simulink model "AUV_ControlsPreliminary"  (R2020b)
settings: Solver=ode23t  StartTime=0.0  StopTime=300  MaxStep=0.01  RelTol=1e-3  EnableMultiTasking=on
PreLoadFcn:
  | AUV_VehicleParameters;
  | Vehicle.Body.markeropacity = 0;
model workspace: external: MATLAB File AUV_DataFile_ORIG.m (data not in the file)
undefined symbols (not defined in the file or in its folder): Environment, Newton, Raphson, smiData, X, x, y, Y, Z
libraries: sm_lib x3123, nesl_utility x51, sharedutil x8, pid_lib x6, AUVCustomPrimitives_Lib x4, shared6dof x1, aerolibasang x1, aerolibadyn x1, SignalEditorBlockLib x1
(part 1 of 62)
settings Model: Creator=cosorio  LastModifiedBy=cosorio
settings DataIOCC: MaxDataPoints=10000  SaveOutput=off  DSMLogging=off  SaveTime=off  SignalLoggingName=logsout_controls
settings OptimizationCC: LifeSpan=inf
settings DebuggingCC: AllowSymbolicDim=off  SFUnexpectedBacktrackingDiag=warning  SFNoUnconditionalDefaultTransitionDiag=warning  SFExecutionAtInitializationDiag=none  ArithmeticOperatorsInVariantConditions=warning
settings SFSimCC: SimUseLocalCustomCode=off  CustomCodeUndefinedFunction=UseInterfaceOnly
settings RTWCC: RTWUseLocalCustomCode=off
settings CodeAppCC: StateflowObjectComments=on
settings GRTTargetCC: TargetLangStandard=C89/C90 (ANSI)
settings ConfigComp: CovMetricSettings=dw  CovSaveCumulativeToWorkspaceVar=on  CovSaveSingleToWorkspaceVar=on  CovExternalEMLEnable=off  CovSFcnEnable=off
settings SimscapeCC: SimscapeLogName=simlog_hydrodynamicsVAR  SimscapeLogLimitData=off  SimscapeLogDataHistory=10000
settings DiagnosticsConfigSet: SimMechanicsUnconnectedFramePorts=none  SimMechanicsConflictingReferenceFrames=none
settings ExplorerConfigSet: InternalSimMechanicsExplorerSettings="<ExplorerConfiguration><canonicalview>aerospace</canonicalview><AnimationSetting><BasePlaybackSpeed>1.0</BasePlaybackSpeed><PlaybackSpeedFactor>4.0</PlaybackSpeedFactor></AnimationSetting><TilePanel><TileInfo><Tiles Columns=\"2\" Count=\"4\" Rows=\"2\"><Column Weight=\"0.4992\"/><Column Weight=\"0.5008\"/><Row Weight=\"0.5\"/><Row Weight=\"0.5\"/><Tile Height=\"1\" Width=\"1\" X=\"0\" Y=\"0\"/><Tile Height=\"1\" Width=\"1\" X=\"0\" Y=\"1\"/><Tile Height=\"1\" Width=\"1\" X=\"1\" Y=\"0\"/><Tile Height=\"1\" Width=\"1\" X=\"1\" Y=\"1\"/></Tiles></TileInfo><SceneInfo><SceneViewer><BGColor><R>1</R><G>1</G><B>1</B></BGColor><Camera><DoPerspective>on</DoPerspective><Position><X>-3.00000146164778636</X><Y>7.03310812635629781e-05</Y><Z>2</Z></Position><Center><X>-1.46164778620002517e-06</X><Y>7.03310812637207838e-05</Y><Z>5</Z></Center><Up><X>0</X><Y>0</Y><Z>-1</Z></Up><ViewLimDist>1</ViewLimDist><YLim>0.466307658154998583</YLim><XLim>0.489133907155592906</XLim></Camera></SceneViewer><SceneViewer><BGColor><R>1</R><G>1</G><B>1</B></BGColor><Camera><DoPerspective>on</DoPerspective><Position><X>-1.46164778620001966e-06</X><Y>7.03310812635620566e-05</Y><Z>2</Z></Position><Center><X>-1.46164778620002517e-06</X><Y>7.03310812637207838e-05</Y><Z>5</Z></Center><Up><X>1</X><Y>0</Y><Z>0</Z></Up><ViewLimDist>1</ViewLimDist><YLim>0.466307658154998583</YLim><XLim>0.489133907155592906</XLim></Camera></SceneViewer><SceneViewer><BGColor><R>1</R><G>1</G><B>1</B></BGColor><Camera><DoPerspective>on</DoPerspective><Position><X>-2.50000146164778636</X><Y>-1.49992966891873625</Y><Z>2.5</Z></Position><Center><X>-1.46164778620002517e-06</X><Y>7.03310812637207838e-05</Y><Z>5</Z></Center><Up><X>0</X><Y>0</Y><Z>-1</Z></Up><ViewLimDist>1</ViewLimDist><YLim>0.466307658154998583</YLim><XLim>0.489133907155592906</XLim></Camera></SceneViewer><SceneViewer><BGColor><R>1</R><G>1</G><B>1</B></BGColor><Camera><DoPerspective>on</DoPerspective><Position><X>-1.46164778620094505e-06</X><Y>-2.99992966891873625</Y><Z>5</Z></Position><Center><X>-1.46164778620002517e-06</X><Y>7.03310812637207838e-05</Y><Z>5</Z></Center><Up><X>0</X><Y>0</Y><Z>-1</Z></Up><ViewLimDist>1</ViewLimDist><YLim>0.466307658154998583</YLim><XLim>0.489133907155592906</XLim></Camera></SceneViewer></SceneInfo></TilePanel><MechEditorPanel><Cameras><Camera><Id>Camera1</Id><Value><Name>Behind</Name><NativeCamera><PositionTrackingFeature>AUV.Muiltibody.Cameras.Behind.R</PositionTrackingFeature><CenterTrackingFeature>AUV.Muiltibody.Cameras.CoM</CenterTrackingFeature><UpVectorTrackingFeature>AUV.Muiltibody.World.W</UpVectorTrackingFeature><CenterTrackingOrigin>on</CenterTrackingOrigin><UpVectorTrackingDirection>-Z</UpVectorTrackingDirection></NativeCamera></Value></Camera><Camera><Id>Camera2</Id><Value><Name>BehindUP</Name><NativeCamera><PositionTrackingFeature>AUV.Muiltibody.Cameras.BehindUP.R</PositionTrackingFeature><CenterTrackingFeature>AUV.Muiltibody.Cameras.CoM</CenterTrackingFeature><UpVectorTrackingFeature>AUV.Muiltibody.World.W</UpVectorTrackingFeature><CenterTrackingOrigin>on</CenterTrackingOrigin><UpVectorTrackingDirection>-Z</UpVectorTrackingDirection></NativeCamera></Value></Camera><Camera><Id>Camera3</Id><Value><Name>BehindDown</Name><NativeCamera><PositionTrackingFeature>AUV.Muiltibody.Cameras.BehindDown.R</PositionTrackingFeature><CenterTrackingFeature>AUV.Muiltibody.Cameras.CoM</CenterTrackingFeature><UpVectorTrackingFeature>AUV.Muiltibody.World.W</UpVectorTrackingFeature><CenterTrackingOrigin>on</CenterTrackingOrigin><UpVectorTrackingDirection>-Z</UpVectorTrackingDirection></NativeCamera></Value></Camera><Camera><Id>Camera4</Id><Value><Name>BehindUPLeft</Name><NativeCamera><PositionTrackingFeature>AUV.Muiltibody.Cameras.BehindUPLeft.R</PositionTrackingFeature><CenterTrackingFeature>AUV.Muiltibody.Cameras.CoM</CenterTrackingFeature><UpVectorTrackingFeature>AUV.Muiltibody.World.W</UpVectorTrackingFeature><CenterTrackingOrigin>on</CenterTrackingOrigin><UpVectorTrackingDirection>-Z</UpVectorTrackingDirection></NativeCamera></Value></Camera><Camera><Id>Camera5</Id><Value><Name>BehindUPRight</Name><NativeCamera><PositionTrackingFeature>AUV.Muiltibody.Cameras.BehindUPRight.R</PositionTrackingFeature><CenterTrackingFeature>AUV.Muiltibody.Cameras.CoM</CenterTrackingFeature><UpVectorTrackingFeature>AUV.Muiltibody.World.W</UpVectorTrackingFeature><CenterTrackingOrigin>on</CenterTrackingOrigin><UpVectorTrackingDirection>-Z</UpVectorTrackingDirection></NativeCamera></Value></Camera><Camera><Id>Camera6</Id><Value><Name>Top</Name><NativeCamera><PositionTrackingFeature>AUV.Muiltibody.Cameras.Top.R</PositionTrackingFeature><CenterTrackingFeature>AUV.Muiltibody.Cameras.CoM</CenterTrackingFeature><UpVectorTrackingFeature>AUV.Muiltibody.World.W</UpVectorTrackingFeature><CenterTrackingOrigin>on</CenterTrackingOrigin><UpVectorTrackingDirection>+X</UpVectorTrackingDirection></NativeCamera></Value></Camera><Camera><Id>Camera7</Id><Value><Name>Side</Name><NativeCamera><PositionTrackingFeature>AUV.Muiltibody.Cameras.Side.R</PositionTrackingFeature><CenterTrackingFeature>AUV.Muiltibody.Cameras.CoM</CenterTrackingFeature><UpVectorTrackingFeature>AUV.Muiltibody.World.W</UpVectorTrackingFeature><CenterTrackingOrigin>on</CenterTrackingOrigin><UpVectorTrackingDirection>-Z</UpVectorTrackingDirection></NativeCamera></Value></Camera><Camera><Id>Camera8</Id><Value><Name>ISO</Name><NativeCamera><PositionTrackingFeature>AUV.Muiltibody.Cameras.ISO.R</PositionTrackingFeature><CenterTrackingFeature>AUV.Muiltibody.Cameras.CoM</CenterTrackingFeature><UpVectorTrackingFeature>AUV.Muiltibody.Cameras.World.W</UpVectorTrackingFeature><CenterTrackingOrigin>on</CenterTrackingOrigin><UpVectorTrackingDirection>-Z</UpVectorTrackingDirection></NativeCamera></Value></Camera></Cameras><GfxPanelCameraMap><MapElement CameraMLId=\"Camera2\" GfxPanelIndex=\"0\"/><MapElement CameraMLId=\"Camera6\" GfxPanelIndex=\"1\"/><MapElement CameraMLId=\"Camera8\" GfxPanelIndex=\"2\"/><MapElement CameraMLId=\"Camera7\" GfxPanelIndex=\"3\"/></GfxPanelCameraMap><VideoCreator><PlaybackSpeedRatio>1.0</PlaybackSpeedRatio><FrameRate>30</FrameRate><VideoFormat>Motion JPEG AVI</VideoFormat><FrameSize>auto</FrameSize></VideoCreator></MechEditorPanel></ExplorerConfiguration>"

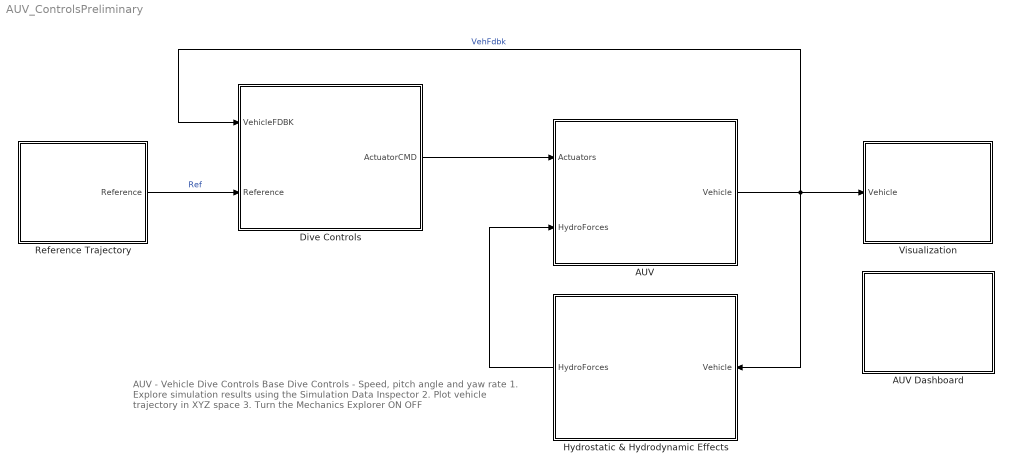
== system AUV_ControlsPreliminary ==
  note: AUV - Vehicle Dive Controls
      | Base Dive Controls - Speed, pitch angle and yaw rate
      |
      | 1. Explore simulation results using the Simulation Data Inspector
      | 2. Plot vehicle trajectory in XYZ space
      | 3. Turn the Mechanics Explorer ON OFF
  AUV : Subsystem  Variant=on  VariantControlMode=label  VariantControl=Choice  LabelModeActiveChoice=Multibody  mask(AUV){VariantLabel=Multibody}
      mask prompts: VariantLabel "Select Variant:"
      mask help:
      | These block contains two variant implementations of the equations of motion for the rigid body dynamics of the underwater vehicle:
      | Multibody Variant  : implements the dynamics using CAD files and Simscape Multibody
      | Singlebody Variant : implements the dynamics using the 6-DoF block from Aerospace Blockset
      mask init:
      | % Set active variant choice for this block
      | if VariantLabel == 1
      |     ActiveChoice = 'Multibody';
      | else
      |     ActiveChoice = 'Singlebody';
      | end
      | 
      | set_param(gcb,'LabelModeActiveChoice',ActiveChoice);
      settings: AttributesFormatString=%<LabelModeActiveChoice>
      mask TypeOptions VariantLabel: Multibody | Singlebody
      mask Display:
      | blk = find_system(gcbh, 'LookUnderMasks', 'all', 'SearchDepth', 1,'FollowLinks','on', 'Parent', gcb,'VariantObject', get_param(gcb,'activevariant'));
      | eval(get_param(blk, 'MaskDisplay'));
  AUV Dashboard : Subsystem
  Dive Controls : Subsystem
  Hydrostatic & Hydrodynamic Effects : Subsystem
      mask Display: image('Drag.png',[0,0.15,1,0.7])
  Reference Trajectory : Subsystem
  Visualization : Subsystem
  wires:
  Hydrostatic & Hydrodynamic Effects/1(HydroForces) -> AUV/2(HydroForces)
  AUV/1(Vehicle) -> Dive Controls/1(VehicleFDBK), Hydrostatic & Hydrodynamic Effects/1(Vehicle), Visualization/1(Vehicle)  "VehFdbk"
  Dive Controls/1(ActuatorCMD) -> AUV/1(Actuators)
  Reference Trajectory/1(Reference) -> Dive Controls/2(Reference)  "Ref"

== system AUV_ControlsPreliminary/AUV ==
  Actuators : Inport
  HydroForces : Inport  Port=2
  Muiltibody : Subsystem  VariantControl=Multibody
      mask Display: image('AUV.png',[0.05,0,0.9,1])
  Singlebody : Subsystem  VariantControl=Singlebody
      mask Display: image('AUVEllipsoid.png',[0.05,0,0.9,1])
  Vehicle : Outport

== system AUV_ControlsPreliminary/AUV Dashboard ==
  note: AUV DASHBOARD
  note: DEPTH (m)x100
  note: DEPTH (cm)
  note: DEPTH (cm)
  note: SPEED
  note: HEADING
  note: HORIZON
  note: VERTICAL SPEED (ft/min)x10
  note: TURN COORDINATOR
  note: DEPTH (ft)x100
  Airspeed Indicator : AirspeedIndicatorBlock  LabelPosition=Hide  ScaleMin=0  ScaleMax=9
  Altimeter : AltimeterBlock  LabelPosition=Hide
  Artificial Horizon : ArtificialHorizonBlock  LabelPosition=Hide
  Climb Rate Indicator : ClimbIndicatorBlock  LabelPosition=Hide
  Heading Indicator : HeadingIndicatorBlock  LabelPosition=Hide
  Turn Coordinator : TurnCoordinatorBlock  LabelPosition=Hide

== system AUV_ControlsPreliminary/Dive Controls ==
  Bus Element In6 : Inport  PortName=VehicleFDBK
  Bus Element In1 : Inport  Port=2  PortName=Reference
  Thrust Controls : Subsystem
  Torque Controls : Subsystem
  Out Bus Element2 : Outport  PortName=ActuatorCMD  Element=Propellers.PPf
  Out Bus Element1 : Outport  PortName=ActuatorCMD  Element=Propellers.PPt
  Out Bus Element4 : Outport  PortName=ActuatorCMD  Element=Propellers.SPf
  Out Bus Element3 : Outport  PortName=ActuatorCMD  Element=Propellers.SPt
  Out Bus Element6 : Outport  PortName=ActuatorCMD  Element=Thrusters.BHTf
  Out Bus Element7 : Outport  PortName=ActuatorCMD  Element=Thrusters.BHTt
  Out Bus Element5 : Outport  PortName=ActuatorCMD  Element=Thrusters.BVTf
  Out Bus Element : Outport  PortName=ActuatorCMD  Element=Thrusters.BVTt
  Out Bus Element8 : Outport  PortName=ActuatorCMD  Element=Thrusters.SHTf
  Out Bus Element9 : Outport  PortName=ActuatorCMD  Element=Thrusters.SHTt
  Out Bus Element10 : Outport  PortName=ActuatorCMD  Element=Thrusters.SVTf
  Out Bus Element11 : Outport  PortName=ActuatorCMD  Element=Thrusters.SVTt
  wires:
  Torque Controls/1(BHTt) -> Out Bus Element7/1
  Torque Controls/2(BVTt) -> Out Bus Element/1
  Torque Controls/3(PPt) -> Out Bus Element1/1
  Torque Controls/4(SPt) -> Out Bus Element3/1
  Torque Controls/5(SHTt) -> Out Bus Element9/1
  Torque Controls/6(SVTt) -> Out Bus Element11/1
  Thrust Controls/3(BVTf) -> Out Bus Element5/1
  Thrust Controls/4(SVTf) -> Out Bus Element10/1
  Thrust Controls/5(BHTf) -> Out Bus Element6/1
  Thrust Controls/6(SHTf) -> Out Bus Element8/1
  Thrust Controls/1(PPf) -> Out Bus Element2/1
  Thrust Controls/2(SPf) -> Out Bus Element4/1
  Bus Element In6/1 -> Thrust Controls/2(VehicleFDBK)
  Bus Element In1/1 -> Thrust Controls/1(Reference)

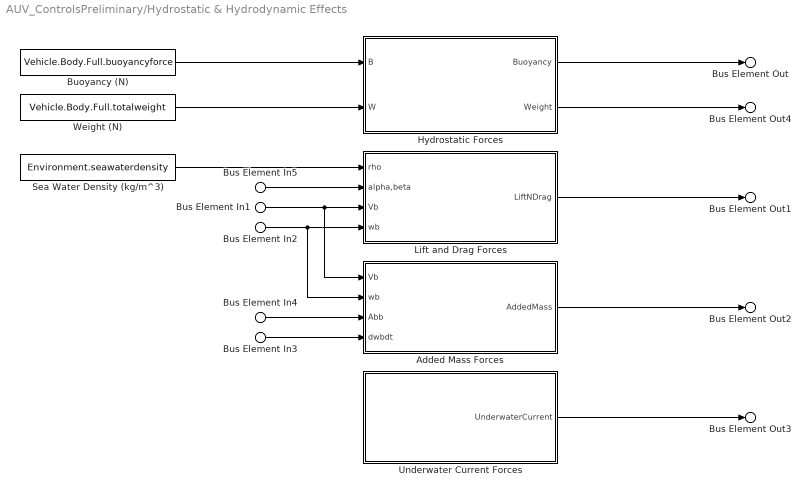
== system AUV_ControlsPreliminary/Hydrostatic & Hydrodynamic Effects ==
  Bus Element In1 : Inport  PortName=Vehicle  Element=CoM.Body.Vb
  Bus Element In2 : Inport  PortName=Vehicle  Element=CoM.Body.wb
  Bus Element In3 : Inport  PortName=Vehicle  Element=CoM.Body.dwbdt
  Bus Element In4 : Inport  PortName=Vehicle  Element=CoM.Derived.Body.Abb
  Bus Element In5 : Inport  PortName=Vehicle  Element=CoM.Derived.Body.Incidences
  Added Mass Forces : Subsystem
  Buoyancy (N) : Constant  Value=Vehicle.Body.Full.buoyancyforce
  Hydrostatic Forces : Subsystem
  Lift and Drag Forces : Subsystem
  Sea Water Density (kg/m^3) : Constant  Value=Environment.seawaterdensity
  Underwater Current Forces : Subsystem
  Weight (N) : Constant  Value=Vehicle.Body.Full.totalweight
  Bus Element Out : Outport  PortName=HydroForces  Element=Buoyancy
  Bus Element Out1 : Outport  PortName=HydroForces  Element=LiftNDrag
  Bus Element Out2 : Outport  PortName=HydroForces  Element=AddedMass
  Bus Element Out3 : Outport  PortName=HydroForces  Element=UnderwaterCurrent
  Bus Element Out4 : Outport  PortName=HydroForces  Element=Weight
  wires:
  Sea Water Density (kg/m^3)/1 -> Lift and Drag Forces/1(rho)
  Bus Element In1/1 -> Lift and Drag Forces/3(Vb), Added Mass Forces/1(Vb)
  Buoyancy (N)/1 -> Hydrostatic Forces/1(B)
  Bus Element In2/1 -> Lift and Drag Forces/4(wb), Added Mass Forces/2(wb)
  Bus Element In4/1 -> Added Mass Forces/3(Abb)
  Bus Element In3/1 -> Added Mass Forces/4(dwbdt)
  Bus Element In5/1 -> Lift and Drag Forces/2(alpha,beta)
  Hydrostatic Forces/1(Buoyancy) -> Bus Element Out/1
  Lift and Drag Forces/1(LiftNDrag) -> Bus Element Out1/1
  Added Mass Forces/1(AddedMass) -> Bus Element Out2/1
  Underwater Current Forces/1(UnderwaterCurrent) -> Bus Element Out3/1
  Weight (N)/1 -> Hydrostatic Forces/2(W)
  Hydrostatic Forces/2(Weight) -> Bus Element Out4/1

== system AUV_ControlsPreliminary/Reference Trajectory ==
  note: NOTE: Double-click on the Reference Trajectory block to choose the different Active Scenario available.
  Reference Trajectory : SignalEditorBlockLib/Signal Editor  FileName=RefTrajectory.mat  ActiveScenario=StraightDiveNTurn  ActiveSignal=Speed  IsBus=off  OutputBusObjectStr=Bus: BusObject  SampleTime=0  OutputAfterFinalValue=Holding final value  Unit=inherit  PreserveSignalName=on
  deg2rad : Gain  Gain=pi/180
  Out Bus Element2 : Outport  PortName=Reference  Element=Speed
  Out Bus Element1 : Outport  PortName=Reference  Element=Depth
  Out Bus Element3 : Outport  PortName=Reference  Element=Heading
  wires:
  Reference Trajectory/1 -> Out Bus Element2/1
  Reference Trajectory/2 -> Out Bus Element1/1
  Reference Trajectory/3 -> deg2rad/1
  deg2rad/1 -> Out Bus Element3/1

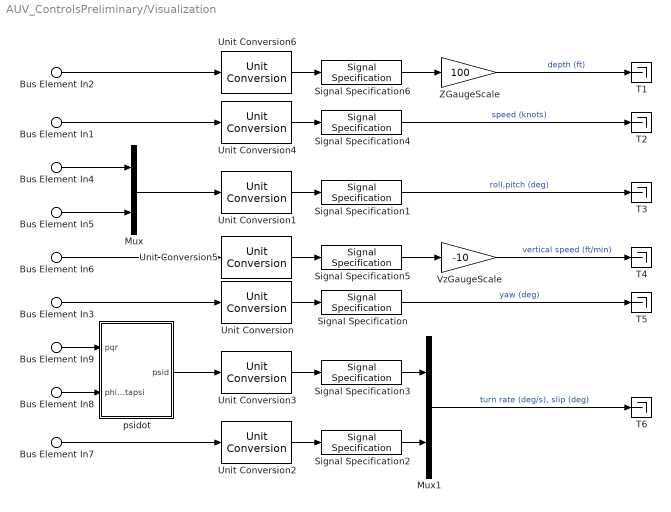
== system AUV_ControlsPreliminary/Visualization ==
  Bus Element In2 : Inport  PortName=Vehicle  Element=CoM.World.Xe.Z
  Bus Element In6 : Inport  PortName=Vehicle  Element=CoM.World.Ve.Vz
  Bus Element In1 : Inport  PortName=Vehicle  Element=CoM.Derived.Body.V
  Bus Element In7 : Inport  PortName=Vehicle  Element=CoM.Derived.Body.Incidences.beta
  Bus Element In8 : Inport  PortName=Vehicle  Element=CoM.Derived.Euler
  Bus Element In3 : Inport  PortName=Vehicle  Element=CoM.Derived.Euler.psi
  Bus Element In4 : Inport  PortName=Vehicle  Element=CoM.Derived.Euler.phi
  Bus Element In5 : Inport  PortName=Vehicle  Element=CoM.Derived.Euler.theta
  Bus Element In9 : Inport  PortName=Vehicle  Element=CoM.Body.wb
  Mux : Mux  Inputs=2
  Mux1 : Mux  Inputs=2
  Signal Specification : SignalSpecification  Unit=deg
  Signal Specification1 : SignalSpecification  Unit=deg
  Signal Specification2 : SignalSpecification  Unit=deg
  Signal Specification3 : SignalSpecification  Unit=deg/s
  Signal Specification4 : SignalSpecification  Unit=kn
  Signal Specification5 : SignalSpecification  Unit=ft/min
  Signal Specification6 : SignalSpecification  Unit=ft
  T{1..6} (6 alike) : Terminator
  Unit Conversion{,1..6} (7 alike) : UnitConversion
  VzGaugeScale : Gain  Gain=-10
  ZGaugeScale : Gain  Gain=100
  psidot : Subsystem
  wires:
  Bus Element In2/1 -> Unit Conversion6/1
  Bus Element In1/1 -> Unit Conversion4/1
  Unit Conversion4/1 -> Signal Specification4/1
  Bus Element In3/1 -> Unit Conversion/1
  Signal Specification/1 -> T5/1  "yaw (deg)"
  Unit Conversion/1 -> Signal Specification/1
  Bus Element In4/1 -> Mux/1
  Bus Element In5/1 -> Mux/2
  Mux/1 -> Unit Conversion1/1
  Unit Conversion1/1 -> Signal Specification1/1
  Signal Specification1/1 -> T3/1  "roll,pitch (deg)"
  Bus Element In6/1 -> Unit Conversion5/1
  Bus Element In7/1 -> Unit Conversion2/1
  Unit Conversion2/1 -> Signal Specification2/1
  Signal Specification2/1 -> Mux1/2
  psidot/1(psid) -> Unit Conversion3/1
  Unit Conversion3/1 -> Signal Specification3/1
  Signal Specification3/1 -> Mux1/1
  Mux1/1 -> T6/1  "turn rate (deg/s), slip (deg)"
  Bus Element In9/1 -> psidot/1(pqr)
  Bus Element In8/1 -> psidot/2(phithetapsi)
  Signal Specification4/1 -> T2/1  "speed (knots)"
  Unit Conversion5/1 -> Signal Specification5/1
  Signal Specification5/1 -> VzGaugeScale/1
  Unit Conversion6/1 -> Signal Specification6/1
  Signal Specification6/1 -> ZGaugeScale/1
  ZGaugeScale/1 -> T1/1  "depth (ft)"
  VzGaugeScale/1 -> T4/1  "vertical speed (ft/min)"

== system AUV_ControlsPreliminary/AUV/Muiltibody ==
  Actuators : Inport
  HydroForces : Inport  Port=2
  6-DOF : sm_lib/Joints/6-DOF Joint  JointMode=Normal  SenseConstraintForce=off  SenseConstraintForceX=off  SenseConstraintForceY=off  SenseConstraintForceZ=off  SenseConstraintTorque=off  SenseConstraintTorqueX=off  SenseConstraintTorqueY=off  SenseConstraintTorqueZ=off  SenseTotalForce=off  SenseTotalForceX=off  SenseTotalForceY=off  SenseTotalForceZ=off  SenseTotalTorque=off  SenseTotalTorqueX=off  SenseTotalTorqueY=off  SenseTotalTorqueZ=off  CompositeWrenchDir=FollowerOnBase  CompositeWrenchFrame=FollowerFrame  PxEquilibriumPosition=0  PxEquilibriumPositionUnits=m  PxSpringStiffness=0  PxSpringStiffnessUnits=N/m  PxDampingCoefficient=0  PxDampingCoefficientUnits=N/(m/s)  PxTorqueActuationMode=NoTorque  PxMotionActuationMode=ComputedMotion  PxSensePosition=off  PxSenseVelocity=off  PxSenseAcceleration=off  PxSenseTorqueForce=off  PxSenseLowerLimitTorqueForce=off  PxSenseUpperLimitTorqueForce=off  PxLowerLimitSpecify=off  PxLowerLimitBound=-1  PxLowerLimitBoundUnits=m  PxLowerLimitStiffness=1e6  PxLowerLimitStiffnessUnits=N/m  PxLowerLimitDamping=1e3  PxLowerLimitDampingUnits=N/(m/s)  PxLowerLimitTransitionRegionWidth=1e-4  PxLowerLimitTransitionRegionWidthUnits=m  PxUpperLimitSpecify=off  PxUpperLimitBound=1  PxUpperLimitBoundUnits=m  PxUpperLimitStiffness=1e6  PxUpperLimitStiffnessUnits=N/m  PxUpperLimitDamping=1e3  PxUpperLimitDampingUnits=N/(m/s)  PxUpperLimitTransitionRegionWidth=1e-4  PxUpperLimitTransitionRegionWidthUnits=m  PxPositionTargetSpecify=off  PxPositionTargetPriority=High  PxPositionTargetValue=0  PxPositionTargetValueUnits=m  PxVelocityTargetSpecify=off  PxVelocityTargetPriority=High  PxVelocityTargetValue=0  PxVelocityTargetValueUnits=m/s  PyEquilibriumPosition=0  PyEquilibriumPositionUnits=m  PySpringStiffness=0  PySpringStiffnessUnits=N/m  PyDampingCoefficient=0  PyDampingCoefficientUnits=N/(m/s)  PyTorqueActuationMode=NoTorque  PyMotionActuationMode=ComputedMotion  PySensePosition=off  PySenseVelocity=off  PySenseAcceleration=off  PySenseTorqueForce=off  PySenseLowerLimitTorqueForce=off  PySenseUpperLimitTorqueForce=off  PyLowerLimitSpecify=off  PyLowerLimitBound=-1  PyLowerLimitBoundUnits=m  PyLowerLimitStiffness=1e6  PyLowerLimitStiffnessUnits=N/m  PyLowerLimitDamping=1e3  PyLowerLimitDampingUnits=N/(m/s)  PyLowerLimitTransitionRegionWidth=1e-4  PyLowerLimitTransitionRegionWidthUnits=m  PyUpperLimitSpecify=off  PyUpperLimitBound=1  PyUpperLimitBoundUnits=m  PyUpperLimitStiffness=1e6  PyUpperLimitStiffnessUnits=N/m  PyUpperLimitDamping=1e3  PyUpperLimitDampingUnits=N/(m/s)  PyUpperLimitTransitionRegionWidth=1e-4  PyUpperLimitTransitionRegionWidthUnits=m  PyPositionTargetSpecify=off  PyPositionTargetPriority=High  PyPositionTargetValue=0  PyPositionTargetValueUnits=m  PyVelocityTargetSpecify=off  PyVelocityTargetPriority=High  PyVelocityTargetValue=0  PyVelocityTargetValueUnits=m/s  PzEquilibriumPosition=0  PzEquilibriumPositionUnits=m  PzSpringStiffness=0  PzSpringStiffnessUnits=N/m  PzDampingCoefficient=0  PzDampingCoefficientUnits=N/(m/s)  PzTorqueActuationMode=NoTorque  PzMotionActuationMode=ComputedMotion  PzSensePosition=off  PzSenseVelocity=off  PzSenseAcceleration=off  PzSenseTorqueForce=off  PzSenseLowerLimitTorqueForce=off  PzSenseUpperLimitTorqueForce=off  PzLowerLimitSpecify=off  PzLowerLimitBound=-1  PzLowerLimitBoundUnits=m  PzLowerLimitStiffness=1e6  PzLowerLimitStiffnessUnits=N/m  PzLowerLimitDamping=1e3  PzLowerLimitDampingUnits=N/(m/s)  PzLowerLimitTransitionRegionWidth=1e-4  PzLowerLimitTransitionRegionWidthUnits=m  PzUpperLimitSpecify=off  PzUpperLimitBound=1  PzUpperLimitBoundUnits=m  PzUpperLimitStiffness=1e6  PzUpperLimitStiffnessUnits=N/m  PzUpperLimitDamping=1e3  PzUpperLimitDampingUnits=N/(m/s)  PzUpperLimitTransitionRegionWidth=1e-4  PzUpperLimitTransitionRegionWidthUnits=m  PzPositionTargetSpecify=on  PzPositionTargetPriority=High  PzPositionTargetValue=Vehicle.InitCond.position(3)  PzPositionTargetValueUnits=m  PzVelocityTargetSpecify=off  PzVelocityTargetPriority=High  PzVelocityTargetValue=0  PzVelocityTargetValueUnits=m/s  SphDefPosRotationMethod=None  SphDefPosRotationAngleUnits=deg  SphDefPosRotationStandardAxis=+Z  SphDefPosRotationAngle=0.0  SphDefPosRotationArbitraryAxis=[0 0 1]  SphDefPosFollAlignAxisA=+X  SphDefPosBaseAlignAxisA=+Y  SphDefPosFollAlignAxisB=+Y  SphDefPosBaseAlignAxisB=+Z  SphDefPosRotationSequenceAxes=FollowerAxes  SphDefPosRotationSequence=XYX  SphDefPosRotationSequenceAngles=[0 0 0]  SphDefPosRotationSequenceAnglesUnits=deg  SphDefPosRotationMatrix=[1 0 0; 0 1 0; 0 0 1]  SphEqPosRotationMethod=None  SphEqPosRotationAngleUnits=deg  SphEqPosRotationStandardAxis=+Z  SphEqPosRotationAngle=0.0  SphEqPosRotationArbitraryAxis=[0 0 1]  SphEqPosFollAlignAxisA=+X  SphEqPosBaseAlignAxisA=+Y  SphEqPosFollAlignAxisB=+Y  SphEqPosBaseAlignAxisB=+Z  SphEqPosRotationSequenceAxes=FollowerAxes  SphEqPosRotationSequence=XYX  SphEqPosRotationSequenceAngles=[0 0 0]  SphEqPosRotationSequenceAnglesUnits=deg  SphEqPosRotationMatrix=[1 0 0; 0 1 0; 0 0 1]  SphSpringStiffness=0  SphSpringStiffnessUnits=N*m/deg  SphDampingCoefficient=0  SphDampingCoefficientUnits=N*m/(deg/s)  SphActuateTorqueX=off  SphActuateTorqueY=off  SphActuateTorqueZ=off  SphActuateTorque=off  SphTorqueActuationMode=NoTorque  SphMotionActuationMode=ComputedMotion  SphActuationFrame=BaseFrame  SphSensePosition=off  SphSenseVelocityX=off  SphSenseVelocityY=off  SphSenseVelocityZ=off  SphSenseVelocity=off  SphSenseAccelerationX=off  SphSenseAccelerationY=off  SphSenseAccelerationZ=off  SphSenseAcceleration=off  SphSenseTorqueX=off  SphSenseTorqueY=off  SphSenseTorqueZ=off  SphSenseTorqueForce=off  SphSenseLowerLimitTorqueMag=off  SphSenseUpperLimitTorqueMag=off  SphSensingFrame=BaseFrame  SphLowerLimitSpecify=off  SphLowerLimitBound=15  SphLowerLimitBoundUnits=deg  SphLowerLimitStiffness=1e4  SphLowerLimitStiffnessUnits=N*m/deg  SphLowerLimitDamping=10  SphLowerLimitDampingUnits=N*m/(deg/s)  SphLowerLimitTransitionRegionWidth=0.1  SphLowerLimitTransitionRegionWidthUnits=deg  SphUpperLimitSpecify=off  SphUpperLimitBound=45  SphUpperLimitBoundUnits=deg  SphUpperLimitStiffness=1e4  SphUpperLimitStiffnessUnits=N*m/deg  SphUpperLimitDamping=10  SphUpperLimitDampingUnits=N*m/(deg/s)  SphUpperLimitTransitionRegionWidth=0.1  SphUpperLimitTransitionRegionWidthUnits=deg  SphPositionTargetRotationMethod=RotationMatrix  SphPositionTargetRotationAngleUnits=deg  SphPositionTargetRotationStandardAxis=+Z  SphPositionTargetRotationAngle=0.0  SphPositionTargetRotationArbitraryAxis=[0 0 1]  SphPositionTargetFollAlignAxisA=+X  SphPositionTargetBaseAlignAxisA=+Y  SphPositionTargetFollAlignAxisB=+Y  SphPositionTargetBaseAlignAxisB=+Z  SphPositionTargetRotationSequenceAxes=BaseAxes  SphPositionTargetRotationSequence=XYX  SphPositionTargetRotationSequenceAngles=[0 0 0]  SphPositionTargetRotationSequenceAnglesUnits=deg  SphPositionTargetRotationMatrix=Vehicle.InitCond.RotMZYX  SphPositionTargetSpecify=on  SphPositionTargetPriority=High  SphVelocityTargetValue=[0 0 0]  SphVelocityTargetValueUnits=deg/s  SphVelocityTargetSpecify=off  SphVelocityTargetPriority=High  SphVelocityTargetInFollowerFrame=on
  AUV Mechanics : Subsystem
      mask Display: image('AUVMechanics.png',[0.05,0.25,0.9,0.5])
  Cameras : Subsystem
  Hydro Forces & Moments : Subsystem
  World : Subsystem
  Vehicle : Outport
  wires:
  AUV Mechanics/1(Vehicle) -> Vehicle/1
  Actuators/1 -> AUV Mechanics/1(Actuators)
  HydroForces/1 -> Hydro Forces & Moments/1(HydroForces)
  connections:
  6-DOF/LConn1 -- World/RConn1
  6-DOF/RConn1 -- Hydro Forces & Moments/RConn1 -- Cameras/RConn1 -- AUV Mechanics/LConn1
  Hydro Forces & Moments/RConn2 -- AUV Mechanics/LConn2

== system AUV_ControlsPreliminary/AUV/Singlebody ==
  Actuators : Inport
  HydroForces : Inport  Port=2
  AUV Mechanics : Subsystem
  Hydro Forces & Moments : Subsystem
  Propellers & Thrusters : Subsystem
  Sum : Sum  Inputs=|++
  Sum1 : Sum  Inputs=++|
  Bus Element Out : Outport  PortName=Vehicle  Element=CoM
  wires:
  HydroForces/1 -> Hydro Forces & Moments/1(HydroForces)
  AUV Mechanics/1(CoM) -> Bus Element Out/1, Hydro Forces & Moments/2(CoM)
  Sum/1 -> AUV Mechanics/1(Fxyz)
  Hydro Forces & Moments/1(Fxyz) -> Sum/2
  Hydro Forces & Moments/2(Mxyz) -> Sum1/2
  Sum1/1 -> AUV Mechanics/2(Mxyz)
  Propellers & Thrusters/1(Fxyz) -> Sum/1
  Propellers & Thrusters/2(Mxyz) -> Sum1/1
  Actuators/1 -> Propellers & Thrusters/1(Actuators)

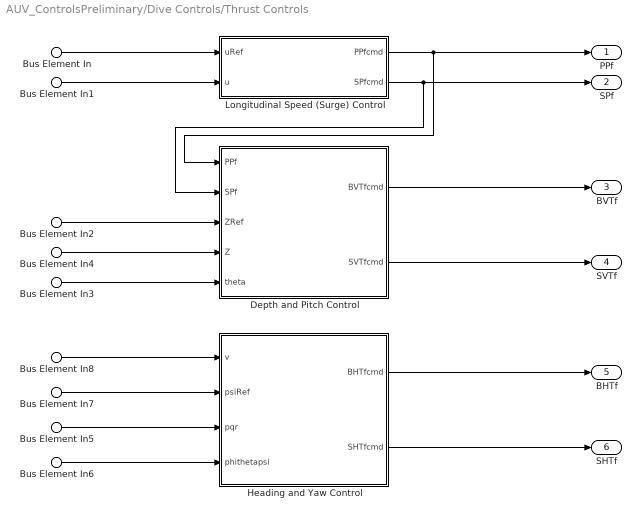
== system AUV_ControlsPreliminary/Dive Controls/Thrust Controls ==
  Bus Element In : Inport  PortName=Reference  Element=Speed
  Bus Element In2 : Inport  PortName=Reference  Element=Depth
  Bus Element In7 : Inport  PortName=Reference  Element=Heading
  Bus Element In1 : Inport  Port=2  PortName=VehicleFDBK  Element=CoM.Body.Vb.u
  Bus Element In8 : Inport  Port=2  PortName=VehicleFDBK  Element=CoM.Body.Vb.v
  Bus Element In5 : Inport  Port=2  PortName=VehicleFDBK  Element=CoM.Body.wb
  Bus Element In6 : Inport  Port=2  PortName=VehicleFDBK  Element=CoM.Derived.Euler
  Bus Element In3 : Inport  Port=2  PortName=VehicleFDBK  Element=CoM.Derived.Euler.theta
  Bus Element In4 : Inport  Port=2  PortName=VehicleFDBK  Element=CoM.World.Xe.Z
  Depth and Pitch Control : Subsystem
  Heading and Yaw Control : Subsystem
  Longitudinal Speed (Surge) Control : Subsystem
  PPf : Outport
  SPf : Outport  Port=2
  BVTf : Outport  Port=3
  SVTf : Outport  Port=4
  BHTf : Outport  Port=5
  SHTf : Outport  Port=6
  wires:
  Longitudinal Speed (Surge) Control/1(PPfcmd) -> Depth and Pitch Control/1(PPf), PPf/1
  Bus Element In/1 -> Longitudinal Speed (Surge) Control/1(uRef)
  Bus Element In1/1 -> Longitudinal Speed (Surge) Control/2(u)
  Longitudinal Speed (Surge) Control/2(SPfcmd) -> Depth and Pitch Control/2(SPf), SPf/1
  Depth and Pitch Control/2(SVTfcmd) -> SVTf/1
  Depth and Pitch Control/1(BVTfcmd) -> BVTf/1
  Heading and Yaw Control/1(BHTfcmd) -> BHTf/1
  Heading and Yaw Control/2(SHTfcmd) -> SHTf/1
  Bus Element In2/1 -> Depth and Pitch Control/3(ZRef)
  Bus Element In3/1 -> Depth and Pitch Control/5(theta)
  Bus Element In4/1 -> Depth and Pitch Control/4(Z)
  Bus Element In5/1 -> Heading and Yaw Control/3(pqr)
  Bus Element In6/1 -> Heading and Yaw Control/4(phithetapsi)
  Bus Element In7/1 -> Heading and Yaw Control/2(psiRef)
  Bus Element In8/1 -> Heading and Yaw Control/1(v)

== system AUV_ControlsPreliminary/Dive Controls/Torque Controls ==
  Tbht (N*m) : Constant  Value=0
  Tbvt (N*m) : Constant  Value=0
  Tpp (N*m) : Constant  Value=0
  Tsht (N*m) : Constant  Value=0
  Tsp (N*m) : Constant  Value=0
  Tsvt (N*m) : Constant  Value=0
  BHTt : Outport
  BVTt : Outport  Port=2
  PPt : Outport  Port=3
  SPt : Outport  Port=4
  SHTt : Outport  Port=5
  SVTt : Outport  Port=6
  wires:
  Tbht (N*m)/1 -> BHTt/1
  Tsvt (N*m)/1 -> SVTt/1
  Tpp (N*m)/1 -> PPt/1
  Tsp (N*m)/1 -> SPt/1
  Tbvt (N*m)/1 -> BVTt/1
  Tsht (N*m)/1 -> SHTt/1

== system AUV_ControlsPreliminary/Hydrostatic & Hydrodynamic Effects/Added Mass Forces ==
  Vb : Inport
  wb : Inport  Port=2
  Abb : Inport  Port=3
  dwbdt : Inport  Port=4
  Added Mass : Subsystem
  Added Mass Matrix : Constant  Value=Vehicle.AddedMass
  Coriolis : Subsystem
  Bus Element Out : Outport  PortName=AddedMass  Element=AMForcesXYZ
  Bus Element Out1 : Outport  PortName=AddedMass  Element=AMMomentsXYZ
  Bus Element Out2 : Outport  PortName=AddedMass  Element=CForcesXYZ
  Bus Element Out3 : Outport  PortName=AddedMass  Element=CMomentsXYZ
  wires:
  Added Mass Matrix/1 -> Added Mass/1(Ma), Coriolis/3(Ma)
  Abb/1 -> Added Mass/2(Abb)
  dwbdt/1 -> Added Mass/3(dwbdt)
  Added Mass/1(Fxyz) -> Bus Element Out/1
  Added Mass/2(Mxyz) -> Bus Element Out1/1
  Vb/1 -> Coriolis/1(Vb)
  wb/1 -> Coriolis/2(wb)
  Coriolis/2(Mxyz) -> Bus Element Out3/1
  Coriolis/1(Fxyz) -> Bus Element Out2/1

== system AUV_ControlsPreliminary/Hydrostatic & Hydrodynamic Effects/Hydrostatic Forces ==
  note: NOTE:
      | The vehicle is assumed to be fully submerged at all times
  B : Inport
  W : Inport  Port=2
  Bus Element Out : Outport  PortName=Buoyancy  Element=BForceZ
  Bus Element Out1 : Outport  Port=2  PortName=Weight  Element=WForceZ
  wires:
  B/1 -> Bus Element Out/1
  W/1 -> Bus Element Out1/1

== system AUV_ControlsPreliminary/Hydrostatic & Hydrodynamic Effects/Lift and Drag Forces ==
  note: NOTE:
      | We are assuming all hydrodynamic coefficients have been
      | computed with respect to the body center of mass, are
      | aligned with the body axes, and were normalized using the
      | front area of the vehicle as reference.
  rho : Inport
  alpha,beta : Inport  Port=2
  Vb : Inport  Port=3
  wb : Inport  Port=4
  CG : Constant  Value=[0,0,0]
  Dynamic Pressure : aerolibasang/Dynamic Pressure
  "Hydrodynamic Forces and Moments " : aerolibadyn/Aerodynamic Forces and Moments   inputAxes=Body  outputForceAxes=Body  outputMomentAxes=Body  S=Vehicle.Body.YZArea  b=Vehicle.Body.hulldiameter  cbar=Vehicle.Body.totallength
  Hydrodynamic Coefficients : Subsystem
  Bus Element Out : Outport  PortName=LiftNDrag  Element=LDForcesXYZ
  Bus Element Out1 : Outport  PortName=LiftNDrag  Element=LDMomentsXYZ
  wires:
  rho/1 -> Dynamic Pressure/2
  Dynamic Pressure/1 -> "Hydrodynamic Forces and Moments "/2
  Vb/1 -> Dynamic Pressure/1, Hydrodynamic Coefficients/3(Vb)
  "Hydrodynamic Forces and Moments "/1 -> Bus Element Out/1
  "Hydrodynamic Forces and Moments "/2 -> Bus Element Out1/1
  CG/1 -> "Hydrodynamic Forces and Moments "/4, "Hydrodynamic Forces and Moments "/3
  alpha,beta/1 -> Hydrodynamic Coefficients/1(alpha,beta)
  wb/1 -> Hydrodynamic Coefficients/2(wb)
  Hydrodynamic Coefficients/1(Coeff) -> "Hydrodynamic Forces and Moments "/1

== system AUV_ControlsPreliminary/Hydrostatic & Hydrodynamic Effects/Underwater Current Forces ==
  note: NOTE:
      | Underwater current velocity is modeled as a first order Markov-like process with a positive
      | time constant m driven by white noise s .
      | Current velocity vector orientation is defined with respect to the World NED reference frame.
  Ground : Ground
  Ground1 : Ground
  Terminator : Terminator
  Terminator1 : Terminator
  Terminator2 : Terminator
  Vcx : Constant  Value=0
  Vcy : Constant  Value=0
  Vcz : Constant  Value=0
  Bus Element Out : Outport  PortName=UnderwaterCurrent  Element=UCForcesXYZ
  Bus Element Out1 : Outport  PortName=UnderwaterCurrent  Element=UCMomentsXYZ
  wires:
  Vcx/1 -> Terminator/1
  Vcy/1 -> Terminator1/1
  Vcz/1 -> Terminator2/1
  Ground/1 -> Bus Element Out/1
  Ground1/1 -> Bus Element Out1/1

== system AUV_ControlsPreliminary/Visualization/psidot ==
  pqr : Inport
  phithetapsi : Inport  Port=2
  Mux1 : Mux  Inputs=[3 3 3]
  psidot : Fcn  Expr=(u[2]*u[4]+u[3]*u[7])/u[8]
  sincos : Trigonometry  Operator=sincos
  psid : Outport  Unit=rad/s  InitialOutput=0  VectorParamsAs1DForOutWhenUnconnected=off
  wires:
  sincos/2 -> Mux1/3
  sincos/1 -> Mux1/2
  phithetapsi/1 -> sincos/1
  pqr/1 -> Mux1/1
  Mux1/1 -> psidot/1
  psidot/1 -> psid/1

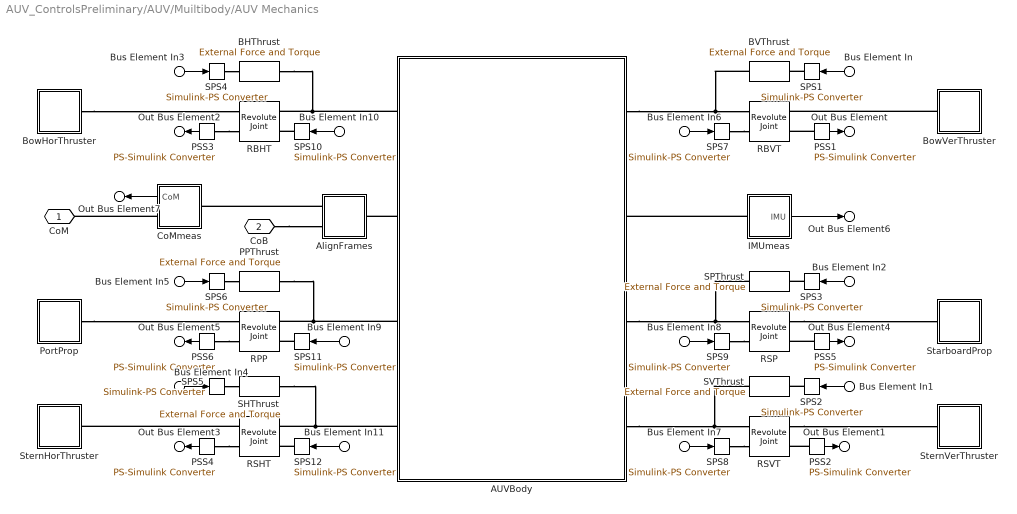
== system AUV_ControlsPreliminary/AUV/Muiltibody/AUV Mechanics ==
  Bus Element In : Inport  PortName=Actuators  Element=Thrusters.BVTf
  Bus Element In1 : Inport  PortName=Actuators  Element=Thrusters.SVTf
  Bus Element In3 : Inport  PortName=Actuators  Element=Thrusters.BHTf
  Bus Element In4 : Inport  PortName=Actuators  Element=Thrusters.SHTf
  Bus Element In6 : Inport  PortName=Actuators  Element=Thrusters.BVTt
  Bus Element In7 : Inport  PortName=Actuators  Element=Thrusters.SVTt
  Bus Element In10 : Inport  PortName=Actuators  Element=Thrusters.BHTt
  Bus Element In11 : Inport  PortName=Actuators  Element=Thrusters.SHTt
  Bus Element In2 : Inport  PortName=Actuators  Element=Propellers.SPf
  Bus Element In5 : Inport  PortName=Actuators  Element=Propellers.PPf
  Bus Element In8 : Inport  PortName=Actuators  Element=Propellers.SPt
  Bus Element In9 : Inport  PortName=Actuators  Element=Propellers.PPt
  AUVBody : Subsystem
      mask Display: image('AUVBody.png');
  AlignFrames : Subsystem
  BHThrust : sm_lib/Forces and Torques/External Force and Torque  ForceResolutionFrame=AttachedFrame  EnableForceX=off  EnableForceY=off  EnableForceZ=on  EnableForce=off  TorqueResolutionFrame=AttachedFrame  EnableTorqueX=off  EnableTorqueY=off  EnableTorqueZ=off  EnableTorque=off
  BVThrust : sm_lib/Forces and Torques/External Force and Torque  ForceResolutionFrame=AttachedFrame  EnableForceX=off  EnableForceY=off  EnableForceZ=on  EnableForce=off  TorqueResolutionFrame=AttachedFrame  EnableTorqueX=off  EnableTorqueY=off  EnableTorqueZ=off  EnableTorque=off
  BowHorThruster : Subsystem
      mask Display: image('TunnelThrusterProp.png',[0.15,0.25,0.7,0.5]);
  BowVerThruster : Subsystem
      mask Display: image('TunnelThrusterProp.png',[0.15,0.25,0.7,0.5]);
  CoMmeas : Subsystem
  IMUmeas : Subsystem
  PPThrust : sm_lib/Forces and Torques/External Force and Torque  ForceResolutionFrame=AttachedFrame  EnableForceX=off  EnableForceY=off  EnableForceZ=on  EnableForce=off  TorqueResolutionFrame=AttachedFrame  EnableTorqueX=off  EnableTorqueY=off  EnableTorqueZ=off  EnableTorque=off
  PSS{1..6} (6 alike) : nesl_utility/PS-Simulink Converter  PhysicalDomain=network_engine_domain  SubClassName=ps_output  LeftPortType=input  RightPortType=output  PseudoPeriodic=off  Frequencies=[]  Unit=rad/s  AffineConversion=off
  PortProp : Subsystem
      mask Display: image('MainProp.png',[0.1,0.1,0.8,0.8]);
  RBHT : sm_lib/Joints/Revolute Joint  JointMode=Normal  SenseConstraintForce=off  SenseConstraintForceX=off  SenseConstraintForceY=off  SenseConstraintForceZ=off  SenseConstraintTorque=off  SenseConstraintTorqueX=off  SenseConstraintTorqueY=off  SenseConstraintTorqueZ=off  SenseTotalForce=off  SenseTotalForceX=off  SenseTotalForceY=off  SenseTotalForceZ=off  SenseTotalTorque=off  SenseTotalTorqueX=off  SenseTotalTorqueY=off  SenseTotalTorqueZ=off  CompositeWrenchDir=FollowerOnBase  CompositeWrenchFrame=BaseFrame  EquilibriumPosition=0  EquilibriumPositionUnits=rad  SpringStiffness=0  SpringStiffnessUnits=N*m/rad  DampingCoefficient=0  DampingCoefficientUnits=N*m/(rad/s)  TorqueActuationMode=InputTorque  MotionActuationMode=ComputedMotion  SensePosition=off  SenseVelocity=on  SenseAcceleration=off  SenseTorqueForce=off  SenseLowerLimitTorqueForce=off  SenseUpperLimitTorqueForce=off  LowerLimitSpecify=off  LowerLimitBound=-90  LowerLimitBoundUnits=deg  LowerLimitStiffness=1e4  LowerLimitStiffnessUnits=N*m/deg  LowerLimitDamping=10  LowerLimitDampingUnits=N*m/(deg/s)  LowerLimitTransitionRegionWidth=0.1  LowerLimitTransitionRegionWidthUnits=deg  UpperLimitSpecify=off  UpperLimitBound=90  UpperLimitBoundUnits=deg  UpperLimitStiffness=1e4  UpperLimitStiffnessUnits=N*m/deg  UpperLimitDamping=10  UpperLimitDampingUnits=N*m/(deg/s)  UpperLimitTransitionRegionWidth=0.1  UpperLimitTransitionRegionWidthUnits=deg  PositionTargetSpecify=on  PositionTargetPriority=Low  PositionTargetValue=smiData.RevoluteJoint(5).Rz.Pos  PositionTargetValueUnits=deg  VelocityTargetSpecify=off  VelocityTargetPriority=High  VelocityTargetValue=0  VelocityTargetValueUnits=deg/s
  RBVT : sm_lib/Joints/Revolute Joint  JointMode=Normal  SenseConstraintForce=off  SenseConstraintForceX=off  SenseConstraintForceY=off  SenseConstraintForceZ=off  SenseConstraintTorque=off  SenseConstraintTorqueX=off  SenseConstraintTorqueY=off  SenseConstraintTorqueZ=off  SenseTotalForce=off  SenseTotalForceX=off  SenseTotalForceY=off  SenseTotalForceZ=off  SenseTotalTorque=off  SenseTotalTorqueX=off  SenseTotalTorqueY=off  SenseTotalTorqueZ=off  CompositeWrenchDir=FollowerOnBase  CompositeWrenchFrame=BaseFrame  EquilibriumPosition=0  EquilibriumPositionUnits=rad  SpringStiffness=0  SpringStiffnessUnits=N*m/rad  DampingCoefficient=0  DampingCoefficientUnits=N*m/(rad/s)  TorqueActuationMode=InputTorque  MotionActuationMode=ComputedMotion  SensePosition=off  SenseVelocity=on  SenseAcceleration=off  SenseTorqueForce=off  SenseLowerLimitTorqueForce=off  SenseUpperLimitTorqueForce=off  LowerLimitSpecify=off  LowerLimitBound=-90  LowerLimitBoundUnits=deg  LowerLimitStiffness=1e4  LowerLimitStiffnessUnits=N*m/deg  LowerLimitDamping=10  LowerLimitDampingUnits=N*m/(deg/s)  LowerLimitTransitionRegionWidth=0.1  LowerLimitTransitionRegionWidthUnits=deg  UpperLimitSpecify=off  UpperLimitBound=90  UpperLimitBoundUnits=deg  UpperLimitStiffness=1e4  UpperLimitStiffnessUnits=N*m/deg  UpperLimitDamping=10  UpperLimitDampingUnits=N*m/(deg/s)  UpperLimitTransitionRegionWidth=0.1  UpperLimitTransitionRegionWidthUnits=deg  PositionTargetSpecify=on  PositionTargetPriority=Low  PositionTargetValue=smiData.RevoluteJoint(2).Rz.Pos  PositionTargetValueUnits=deg  VelocityTargetSpecify=off  VelocityTargetPriority=High  VelocityTargetValue=0  VelocityTargetValueUnits=deg/s
  RPP : sm_lib/Joints/Revolute Joint  JointMode=Normal  SenseConstraintForce=off  SenseConstraintForceX=off  SenseConstraintForceY=off  SenseConstraintForceZ=off  SenseConstraintTorque=off  SenseConstraintTorqueX=off  SenseConstraintTorqueY=off  SenseConstraintTorqueZ=off  SenseTotalForce=off  SenseTotalForceX=off  SenseTotalForceY=off  SenseTotalForceZ=off  SenseTotalTorque=off  SenseTotalTorqueX=off  SenseTotalTorqueY=off  SenseTotalTorqueZ=off  CompositeWrenchDir=FollowerOnBase  CompositeWrenchFrame=BaseFrame  EquilibriumPosition=0  EquilibriumPositionUnits=rad  SpringStiffness=0  SpringStiffnessUnits=N*m/rad  DampingCoefficient=0  DampingCoefficientUnits=N*m/(rad/s)  TorqueActuationMode=InputTorque  MotionActuationMode=ComputedMotion  SensePosition=off  SenseVelocity=on  SenseAcceleration=off  SenseTorqueForce=off  SenseLowerLimitTorqueForce=off  SenseUpperLimitTorqueForce=off  LowerLimitSpecify=off  LowerLimitBound=-90  LowerLimitBoundUnits=deg  LowerLimitStiffness=1e4  LowerLimitStiffnessUnits=N*m/deg  LowerLimitDamping=10  LowerLimitDampingUnits=N*m/(deg/s)  LowerLimitTransitionRegionWidth=0.1  LowerLimitTransitionRegionWidthUnits=deg  UpperLimitSpecify=off  UpperLimitBound=90  UpperLimitBoundUnits=deg  UpperLimitStiffness=1e4  UpperLimitStiffnessUnits=N*m/deg  UpperLimitDamping=10  UpperLimitDampingUnits=N*m/(deg/s)  UpperLimitTransitionRegionWidth=0.1  UpperLimitTransitionRegionWidthUnits=deg  PositionTargetSpecify=on  PositionTargetPriority=Low  PositionTargetValue=smiData.RevoluteJoint(4).Rz.Pos  PositionTargetValueUnits=deg  VelocityTargetSpecify=off  VelocityTargetPriority=High  VelocityTargetValue=0  VelocityTargetValueUnits=deg/s
  RSHT : sm_lib/Joints/Revolute Joint  JointMode=Normal  SenseConstraintForce=off  SenseConstraintForceX=off  SenseConstraintForceY=off  SenseConstraintForceZ=off  SenseConstraintTorque=off  SenseConstraintTorqueX=off  SenseConstraintTorqueY=off  SenseConstraintTorqueZ=off  SenseTotalForce=off  SenseTotalForceX=off  SenseTotalForceY=off  SenseTotalForceZ=off  SenseTotalTorque=off  SenseTotalTorqueX=off  SenseTotalTorqueY=off  SenseTotalTorqueZ=off  CompositeWrenchDir=FollowerOnBase  CompositeWrenchFrame=BaseFrame  EquilibriumPosition=0  EquilibriumPositionUnits=rad  SpringStiffness=0  SpringStiffnessUnits=N*m/rad  DampingCoefficient=0  DampingCoefficientUnits=N*m/(rad/s)  TorqueActuationMode=InputTorque  MotionActuationMode=ComputedMotion  SensePosition=off  SenseVelocity=on  SenseAcceleration=off  SenseTorqueForce=off  SenseLowerLimitTorqueForce=off  SenseUpperLimitTorqueForce=off  LowerLimitSpecify=off  LowerLimitBound=-90  LowerLimitBoundUnits=deg  LowerLimitStiffness=1e4  LowerLimitStiffnessUnits=N*m/deg  LowerLimitDamping=10  LowerLimitDampingUnits=N*m/(deg/s)  LowerLimitTransitionRegionWidth=0.1  LowerLimitTransitionRegionWidthUnits=deg  UpperLimitSpecify=off  UpperLimitBound=90  UpperLimitBoundUnits=deg  UpperLimitStiffness=1e4  UpperLimitStiffnessUnits=N*m/deg  UpperLimitDamping=10  UpperLimitDampingUnits=N*m/(deg/s)  UpperLimitTransitionRegionWidth=0.1  UpperLimitTransitionRegionWidthUnits=deg  PositionTargetSpecify=on  PositionTargetPriority=Low  PositionTargetValue=smiData.RevoluteJoint(6).Rz.Pos  PositionTargetValueUnits=deg  VelocityTargetSpecify=off  VelocityTargetPriority=High  VelocityTargetValue=0  VelocityTargetValueUnits=deg/s
  RSP : sm_lib/Joints/Revolute Joint  JointMode=Normal  SenseConstraintForce=off  SenseConstraintForceX=off  SenseConstraintForceY=off  SenseConstraintForceZ=off  SenseConstraintTorque=off  SenseConstraintTorqueX=off  SenseConstraintTorqueY=off  SenseConstraintTorqueZ=off  SenseTotalForce=off  SenseTotalForceX=off  SenseTotalForceY=off  SenseTotalForceZ=off  SenseTotalTorque=off  SenseTotalTorqueX=off  SenseTotalTorqueY=off  SenseTotalTorqueZ=off  CompositeWrenchDir=FollowerOnBase  CompositeWrenchFrame=BaseFrame  EquilibriumPosition=0  EquilibriumPositionUnits=rad  SpringStiffness=0  SpringStiffnessUnits=N*m/rad  DampingCoefficient=0  DampingCoefficientUnits=N*m/(rad/s)  TorqueActuationMode=InputTorque  MotionActuationMode=ComputedMotion  SensePosition=off  SenseVelocity=on  SenseAcceleration=off  SenseTorqueForce=off  SenseLowerLimitTorqueForce=off  SenseUpperLimitTorqueForce=off  LowerLimitSpecify=off  LowerLimitBound=-90  LowerLimitBoundUnits=deg  LowerLimitStiffness=1e4  LowerLimitStiffnessUnits=N*m/deg  LowerLimitDamping=10  LowerLimitDampingUnits=N*m/(deg/s)  LowerLimitTransitionRegionWidth=0.1  LowerLimitTransitionRegionWidthUnits=deg  UpperLimitSpecify=off  UpperLimitBound=90  UpperLimitBoundUnits=deg  UpperLimitStiffness=1e4  UpperLimitStiffnessUnits=N*m/deg  UpperLimitDamping=10  UpperLimitDampingUnits=N*m/(deg/s)  UpperLimitTransitionRegionWidth=0.1  UpperLimitTransitionRegionWidthUnits=deg  PositionTargetSpecify=on  PositionTargetPriority=Low  PositionTargetValue=smiData.RevoluteJoint(1).Rz.Pos  PositionTargetValueUnits=deg  VelocityTargetSpecify=off  VelocityTargetPriority=High  VelocityTargetValue=0  VelocityTargetValueUnits=deg/s
  RSVT : sm_lib/Joints/Revolute Joint  JointMode=Normal  SenseConstraintForce=off  SenseConstraintForceX=off  SenseConstraintForceY=off  SenseConstraintForceZ=off  SenseConstraintTorque=off  SenseConstraintTorqueX=off  SenseConstraintTorqueY=off  SenseConstraintTorqueZ=off  SenseTotalForce=off  SenseTotalForceX=off  SenseTotalForceY=off  SenseTotalForceZ=off  SenseTotalTorque=off  SenseTotalTorqueX=off  SenseTotalTorqueY=off  SenseTotalTorqueZ=off  CompositeWrenchDir=FollowerOnBase  CompositeWrenchFrame=BaseFrame  EquilibriumPosition=0  EquilibriumPositionUnits=rad  SpringStiffness=0  SpringStiffnessUnits=N*m/rad  DampingCoefficient=0  DampingCoefficientUnits=N*m/(rad/s)  TorqueActuationMode=InputTorque  MotionActuationMode=ComputedMotion  SensePosition=off  SenseVelocity=on  SenseAcceleration=off  SenseTorqueForce=off  SenseLowerLimitTorqueForce=off  SenseUpperLimitTorqueForce=off  LowerLimitSpecify=off  LowerLimitBound=-90  LowerLimitBoundUnits=deg  LowerLimitStiffness=1e4  LowerLimitStiffnessUnits=N*m/deg  LowerLimitDamping=10  LowerLimitDampingUnits=N*m/(deg/s)  LowerLimitTransitionRegionWidth=0.1  LowerLimitTransitionRegionWidthUnits=deg  UpperLimitSpecify=off  UpperLimitBound=90  UpperLimitBoundUnits=deg  UpperLimitStiffness=1e4  UpperLimitStiffnessUnits=N*m/deg  UpperLimitDamping=10  UpperLimitDampingUnits=N*m/(deg/s)  UpperLimitTransitionRegionWidth=0.1  UpperLimitTransitionRegionWidthUnits=deg  PositionTargetSpecify=on  PositionTargetPriority=Low  PositionTargetValue=smiData.RevoluteJoint(3).Rz.Pos  PositionTargetValueUnits=deg  VelocityTargetSpecify=off  VelocityTargetPriority=High  VelocityTargetValue=0  VelocityTargetValueUnits=deg/s
  SHThrust : sm_lib/Forces and Torques/External Force and Torque  ForceResolutionFrame=AttachedFrame  EnableForceX=off  EnableForceY=off  EnableForceZ=on  EnableForce=off  TorqueResolutionFrame=AttachedFrame  EnableTorqueX=off  EnableTorqueY=off  EnableTorqueZ=off  EnableTorque=off
  SPS{1..6} (6 alike) : nesl_utility/Simulink-PS Converter  PhysicalDomain=network_engine_domain  SubClassName=ps_input  LeftPortType=input  RightPortType=output  PseudoPeriodic=off  Frequencies=[]  NoiseDistribution=none  NoiseParameters=[]  Unit=N  AffineConversion=off  FilteringAndDerivatives=provide  SimscapeFilterOrder=1  InputFilterTimeConstant=0.001  UdotUserProvided=0
  SPS{7..12} (6 alike) : nesl_utility/Simulink-PS Converter  PhysicalDomain=network_engine_domain  SubClassName=ps_input  LeftPortType=input  RightPortType=output  PseudoPeriodic=off  Frequencies=[]  NoiseDistribution=none  NoiseParameters=[]  Unit=N*m  AffineConversion=off  FilteringAndDerivatives=provide  SimscapeFilterOrder=1  InputFilterTimeConstant=0.001  UdotUserProvided=0
  SPThrust : sm_lib/Forces and Torques/External Force and Torque  ForceResolutionFrame=AttachedFrame  EnableForceX=off  EnableForceY=off  EnableForceZ=on  EnableForce=off  TorqueResolutionFrame=AttachedFrame  EnableTorqueX=off  EnableTorqueY=off  EnableTorqueZ=off  EnableTorque=off
  SVThrust : sm_lib/Forces and Torques/External Force and Torque  ForceResolutionFrame=AttachedFrame  EnableForceX=off  EnableForceY=off  EnableForceZ=on  EnableForce=off  TorqueResolutionFrame=AttachedFrame  EnableTorqueX=off  EnableTorqueY=off  EnableTorqueZ=off  EnableTorque=off
  StarboardProp : Subsystem
      mask Display: image('MainProp.png',[0.1,0.1,0.8,0.8]);
  SternHorThruster : Subsystem
      mask Display: image('TunnelThrusterProp.png',[0.15,0.25,0.7,0.5]);
  SternVerThruster : Subsystem
      mask Display: image('TunnelThrusterProp.png',[0.15,0.25,0.7,0.5]);
  CoM : PMIOPort  Side=Left
  CoB : PMIOPort  Port=2  Side=Left
  Out Bus Element6 : Outport  PortName=Vehicle  Element=IMU
  Out Bus Element4 : Outport  PortName=Vehicle  Element=Propellers.SPw
  Out Bus Element5 : Outport  PortName=Vehicle  Element=Propellers.PPw
  Out Bus Element : Outport  PortName=Vehicle  Element=Thrusters.BVTw
  Out Bus Element1 : Outport  PortName=Vehicle  Element=Thrusters.SVTw
  Out Bus Element2 : Outport  PortName=Vehicle  Element=Thrusters.BHTw
  Out Bus Element3 : Outport  PortName=Vehicle  Element=Thrusters.SHTw
  Out Bus Element7 : Outport  PortName=Vehicle  Element=CoM
  wires:
  PSS1/1 -> Out Bus Element/1
  PSS2/1 -> Out Bus Element1/1
  PSS3/1 -> Out Bus Element2/1
  PSS4/1 -> Out Bus Element3/1
  PSS5/1 -> Out Bus Element4/1
  PSS6/1 -> Out Bus Element5/1
  IMUmeas/1(IMU) -> Out Bus Element6/1
  Bus Element In/1 -> SPS1/1
  Bus Element In1/1 -> SPS2/1
  Bus Element In2/1 -> SPS3/1
  Bus Element In3/1 -> SPS4/1
  Bus Element In4/1 -> SPS5/1
  Bus Element In5/1 -> SPS6/1
  CoMmeas/1(CoM) -> Out Bus Element7/1
  Bus Element In6/1 -> SPS7/1
  Bus Element In7/1 -> SPS8/1
  Bus Element In8/1 -> SPS9/1
  Bus Element In9/1 -> SPS11/1
  Bus Element In10/1 -> SPS10/1
  Bus Element In11/1 -> SPS12/1
  connections:
  PortProp/LConn1 -- RPP/RConn1
  AUVBody/LConn1 -- BHThrust/RConn1 -- RBHT/LConn1
  AUVBody/LConn4 -- SHThrust/RConn1 -- RSHT/LConn1
  BowVerThruster/LConn1 -- RBVT/RConn1
  RSP/RConn1 -- StarboardProp/LConn1
  AUVBody/RConn4 -- RSVT/LConn1 -- SVThrust/RConn1
  BowHorThruster/LConn1 -- RBHT/RConn1
  RSVT/RConn1 -- SternVerThruster/LConn1
  AUVBody/RConn1 -- RBVT/LConn1 -- BVThrust/RConn1
  AUVBody/RConn3 -- RSP/LConn1 -- SPThrust/RConn1
  RSHT/RConn1 -- SternHorThruster/LConn1
  AUVBody/LConn3 -- PPThrust/RConn1 -- RPP/LConn1
  AUVBody/LConn2 -- AlignFrames/RConn1
  PSS1/LConn1 -- RBVT/RConn2
  PSS2/LConn1 -- RSVT/RConn2
  PSS3/LConn1 -- RBHT/RConn2
  PSS4/LConn1 -- RSHT/RConn2
  PSS5/LConn1 -- RSP/RConn2
  PSS6/LConn1 -- RPP/RConn2
  IMUmeas/LConn1 -- AUVBody/RConn2
  SPS1/RConn1 -- BVThrust/LConn1
  SPS2/RConn1 -- SVThrust/LConn1
  SPS3/RConn1 -- SPThrust/LConn1
  SPS4/RConn1 -- BHThrust/LConn1
  SPS5/RConn1 -- SHThrust/LConn1
  SPS6/RConn1 -- PPThrust/LConn1
  AlignFrames/LConn1 -- CoMmeas/LConn1
  CoMmeas/RConn1 -- CoM/RConn1
  SPS7/RConn1 -- RBVT/LConn2
  SPS8/RConn1 -- RSVT/LConn2
  SPS9/RConn1 -- RSP/LConn2
  SPS10/RConn1 -- RBHT/LConn2
  SPS11/RConn1 -- RPP/LConn2
  SPS12/RConn1 -- RSHT/LConn2
  CoB/RConn1 -- AlignFrames/LConn2
